simulink model "task4"  (R2018b)
settings: Solver=VariableStepAuto  StartTime=0.0  StopTime=5348  RelTol=1e-3
undefined symbols (not defined in the file): Ion, Lithium
libraries: powerlib x24, powerlib_meascontrol x6, electricdrivelib x4, pePwmGenerator x4, aerolibanimutils x1
settings Model: Creator=ibrahim yosry  LastModifiedBy=ibrahim yosry
settings SolverCC: ZeroCrossAlgorithm=Adaptive
settings DebuggingCC: IgnoredZcDiagnostic=none  LibraryContextMissingDiagnostic=none
settings SFSimCC: SimUseLocalCustomCode=off
settings RTWCC: RTWUseLocalCustomCode=off

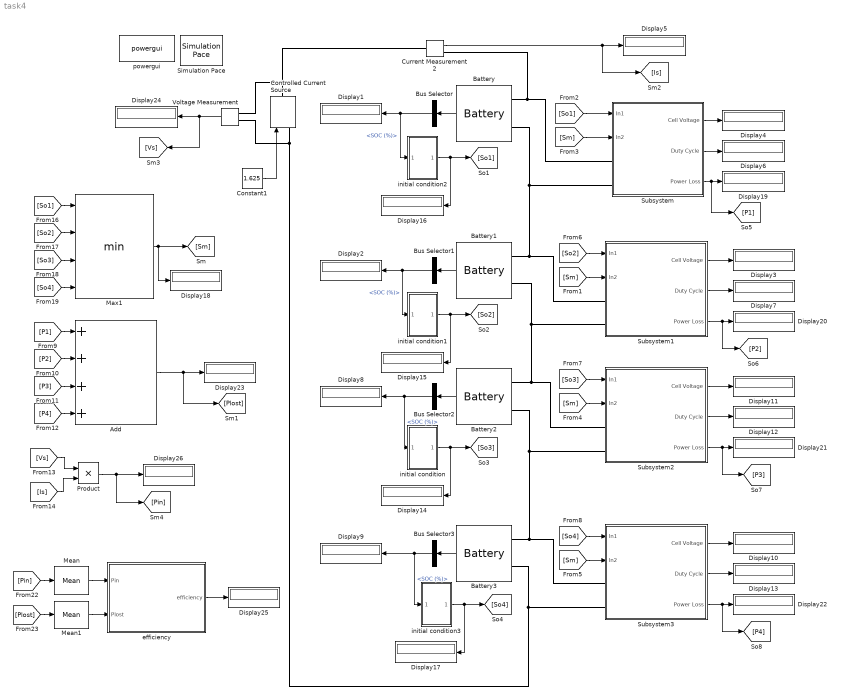
== system task4 ==
  Add : Sum  Inputs=++++
  Battery : electricdrivelib/Extra Sources/Battery  BatType=Lithium-Ion  ShowTempParam=off  ThermalPreset=no  ShowAgeParam=off  NomV=3.6  NomQ=3.4  SOC=14  Batt_Tr=30  PresetModel=on  MaxQ=3.4  MinV=2.7  FullV=4.1904  Dis_rate=1.4783  R=0.010588  Normal_OP=3.0748  expZone="[3.8894     0.16704]"  current=[6.5 13 32.5]  Units=Time  Tci=20  NomT=20  T2=-30  MaxQ2=4.8  FullV2=7.1  Normal_OP2=5.655  expZone2="[6.58           1]"  Rca=0.6  ti=2000  Dp=0  Neq0=0  Tsim=1e6  Ta1=25  Qeol=5.4*0.9  Reol=0.013333*1.2  Char_age=[2.3478, 3]  Dis_age=[2.3478, 10]  N1=1500  N2=10500  N3=1000  N4=1400  Ta2=45  N5=950
      settings: SourceProductName=Simscape Electrical
  Battery1 : electricdrivelib/Extra Sources/Battery  BatType=Lithium-Ion  ShowTempParam=off  ThermalPreset=no  ShowAgeParam=off  NomV=3.6  NomQ=3.4  SOC=24  Batt_Tr=30  PresetModel=on  MaxQ=3.4  MinV=2.7  FullV=4.1904  Dis_rate=1.4783  R=0.010588  Normal_OP=3.0748  expZone="[3.8894     0.16704]"  current=[6.5 13 32.5]  Units=Time  Tci=20  NomT=20  T2=-30  MaxQ2=4.8  FullV2=7.1  Normal_OP2=5.655  expZone2="[6.58           1]"  Rca=0.6  ti=2000  Dp=0  Neq0=0  Tsim=1e6  Ta1=25  Qeol=5.4*0.9  Reol=0.013333*1.2  Char_age=[2.3478, 3]  Dis_age=[2.3478, 10]  N1=1500  N2=10500  N3=1000  N4=1400  Ta2=45  N5=950
      settings: SourceProductName=Simscape Electrical
  Battery2 : electricdrivelib/Extra Sources/Battery  BatType=Lithium-Ion  ShowTempParam=off  ThermalPreset=no  ShowAgeParam=off  NomV=3.6  NomQ=3.4  SOC=30  Batt_Tr=30  PresetModel=on  MaxQ=3.4  MinV=2.7  FullV=4.1904  Dis_rate=1.4783  R=0.010588  Normal_OP=3.0748  expZone="[3.8894     0.16704]"  current=[6.5 13 32.5]  Units=Time  Tci=20  NomT=20  T2=-30  MaxQ2=4.8  FullV2=7.1  Normal_OP2=5.655  expZone2="[6.58           1]"  Rca=0.6  ti=2000  Dp=0  Neq0=0  Tsim=1e6  Ta1=25  Qeol=5.4*0.9  Reol=0.013333*1.2  Char_age=[2.3478, 3]  Dis_age=[2.3478, 10]  N1=1500  N2=10500  N3=1000  N4=1400  Ta2=45  N5=950
      settings: SourceProductName=Simscape Electrical
  Battery3 : electricdrivelib/Extra Sources/Battery  BatType=Lithium-Ion  ShowTempParam=off  ThermalPreset=no  ShowAgeParam=off  NomV=3.6  NomQ=3.4  SOC=45  Batt_Tr=30  PresetModel=on  MaxQ=3.4  MinV=2.7  FullV=4.1904  Dis_rate=1.4783  R=0.010588  Normal_OP=3.0748  expZone="[3.8894     0.16704]"  current=[6.5 13 32.5]  Units=Time  Tci=20  NomT=20  T2=-30  MaxQ2=4.8  FullV2=7.1  Normal_OP2=5.655  expZone2="[6.58           1]"  Rca=0.6  ti=2000  Dp=0  Neq0=0  Tsim=1e6  Ta1=25  Qeol=5.4*0.9  Reol=0.013333*1.2  Char_age=[2.3478, 3]  Dis_age=[2.3478, 10]  N1=1500  N2=10500  N3=1000  N4=1400  Ta2=45  N5=950
      settings: SourceProductName=Simscape Electrical
  Bus Selector{,1..3} (4 alike) : BusSelector  OutputSignals=SOC (%)
  Constant1 : Constant  Value=1.625
  Controlled Current Source : powerlib/Electrical Sources/Controlled Current Source  Initialize=on  Source_Type=DC  Amplitude=1.625  Phase=0  Frequency=0  Measurements=None
      settings: SourceProductName=Simscape Electrical
  Current Measurement2 : powerlib/Measurements/Current Measurement  PhasorSimulation=off  OutputType=Complex  PSBequivalent=0
      settings: SourceProductName=Simscape Electrical
  Display{1..26} (26 alike) : Display
  Max1 : MinMax  Inputs=4  ZeroCross=off
  Mean : powerlib_meascontrol/Measurements/Mean  Freq=1/1000  Vinit=0  Ts=0
  Mean1 : powerlib_meascontrol/Measurements/Mean  Freq=1/1000  Vinit=0  Ts=0
  Product : Product
  Simulation Pace : aerolibanimutils/Simulation Pace  SimulationPace=100  SleepMode=MATLAB Thread  OutputPaceError=off  SampleTime=1/30
  Subsystem : Subsystem
  Subsystem1 : Subsystem
  Subsystem2 : Subsystem
  Subsystem3 : Subsystem
  Voltage Measurement : powerlib/Measurements/Voltage Measurement  PhasorSimulation=off  OutputType=Complex  PSBequivalent=0
      settings: SourceProductName=Simscape Electrical
  efficiency : MATLAB Function  TreatAsAtomicUnit=on
  initial condition : Subsystem
      mask Display: image('F:\hima\zpEWIvRg.jpg');
  initial condition1 : Subsystem
      mask Display: image('F:\hima\zpEWIvRg.jpg');
  initial condition2 : Subsystem
      mask Display: image('F:\hima\zpEWIvRg.jpg');
  initial condition3 : Subsystem
      mask Display: image('F:\hima\zpEWIvRg.jpg');
  powergui : powerlib/powergui  Priority=1  SimulationMode=Continuous  SampleTime=50e-6  frequency=60  Iterations=50  frequencyindice=0  Pbase=100e6  ErrMax=1e-4  UnitsV=kV  UnitsW=MW  buscounter=0  FunctionMessages=off  echomessages=off  EnableUseOfTLC=off  CurrentSourceSwitches=off  DisableSnubberDevices=off  DisableRonSwitches=off  DisableVfSwitches=off  DisplayEquations=off  SolverType=Tustin/Backward Euler (TBE)  Interpol=off  ExternalGateDelay=off  methode=off  Ts=100  x0status=blocks  SPID=on  SwTol=0  HookPort=off  RestoreLinks=warning  ResistiveCurrentMeasurement=off  Frange=[0:2:500]  Ylog=off  Xlog=on  ShowGrid=off  save=off  variable=ZData  structure=0  ZoomFFT=off  StartTime=0.0  cycles=1  DisplayStyle=1  fundamental=60  FreqAxis=off  MaxFrequency=1000  frequencyindicesteady=1  RmsSteady=1  display=off
  wires:
  Bus Selector/1 -> initial condition2/1(<SOC (%)>), Display1/1  "<SOC (%)>"
  Constant1/1 -> Controlled Current Source/1
  Current Measurement2/1 -> [Is], Display5/1
  Battery/1 -> Bus Selector/1
  Subsystem/1(Cell Voltage) -> Display4/1
  Subsystem/2(Duty Cycle) -> Display6/1
  Subsystem1/1(Cell Voltage) -> Display3/1
  Subsystem1/2(Duty Cycle) -> Display7/1
  Battery1/1 -> Bus Selector1/1
  Bus Selector1/1 -> initial condition1/1(<SOC (%)>), Display2/1  "<SOC (%)>"
  Bus Selector3/1 -> initial condition3/1(<SOC (%)>), Display9/1  "<SOC (%)>"
  Subsystem2/2(Duty Cycle) -> Display12/1
  Subsystem3/1(Cell Voltage) -> Display10/1
  Battery3/1 -> Bus Selector3/1
  Subsystem2/1(Cell Voltage) -> Display11/1
  Subsystem3/2(Duty Cycle) -> Display13/1
  Battery2/1 -> Bus Selector2/1
  Bus Selector2/1 -> initial condition/1(<SOC (%)>), Display8/1  "<SOC (%)>"
  initial condition/1(Out1) -> [So3], Display14/1
  initial condition1/1(Out1) -> [So2], Display15/1
  initial condition2/1(Out1) -> [So1], Display16/1
  initial condition3/1(Out1) -> [So4], Display17/1
  [So2] -> Max1/2
  [So1] -> Max1/1
  Max1/1 -> [Sm], Display18/1
  [So3] -> Max1/3
  [So4] -> Max1/4
  [So1] -> Subsystem/1(In1)
  [Sm] -> Subsystem/2(In2)
  [Sm] -> Subsystem1/2(In2)
  [Sm] -> Subsystem2/2(In2)
  [Sm] -> Subsystem3/2(In2)
  [So2] -> Subsystem1/1(In1)
  [So3] -> Subsystem2/1(In1)
  [So4] -> Subsystem3/1(In1)
  Subsystem/3(Power Loss) -> Display19/1, [P1]
  Subsystem1/3(Power Loss) -> Display20/1, [P2]
  Subsystem2/3(Power Loss) -> Display21/1, [P3]
  Subsystem3/3(Power Loss) -> Display22/1, [P4]
  [P4] -> Add/4
  [P2] -> Add/2
  [P1] -> Add/1
  [P3] -> Add/3
  Voltage Measurement/1 -> Display24/1, [Vs]
  [Vs] -> Product/1
  [Is] -> Product/2
  efficiency/1(efficiency) -> Display25/1
  Product/1 -> Display26/1, [Pin]
  Add/1 -> Display23/1, [Plost]
  [Pin] -> Mean/1
  Mean/1 -> efficiency/1(Pin)
  Mean1/1 -> efficiency/2(Plost)
  [Plost] -> Mean1/1
  connections:
  Current Measurement2/LConn1 -- Controlled Current Source/RConn1 -- Voltage Measurement/LConn1
  Battery/LConn1 -- Current Measurement2/RConn1 -- Subsystem/LConn1
  Subsystem1/LConn1 -- Battery/LConn2 -- Subsystem/LConn2 -- Battery1/LConn1
  Subsystem2/LConn1 -- Battery1/LConn2 -- Subsystem1/LConn2 -- Battery2/LConn1
  Subsystem2/LConn2 -- Battery3/LConn1 -- Subsystem3/LConn1 -- Battery2/LConn2
  Subsystem3/LConn2 -- Controlled Current Source/LConn1 -- Voltage Measurement/LConn2 -- Battery3/LConn2

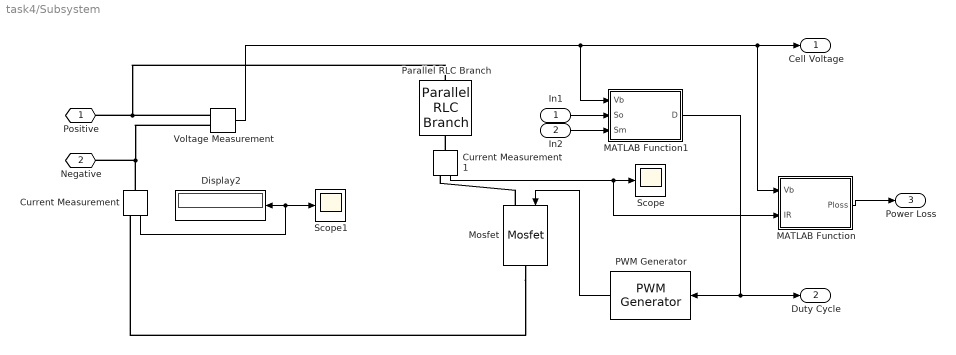
== system task4/Subsystem ==
  In1 : Inport
  In2 : Inport  Port=2
  Current Measurement : powerlib/Measurements/Current Measurement  PhasorSimulation=off  OutputType=Complex  PSBequivalent=0
      settings: SourceProductName=Simscape Electrical
  Current Measurement1 : powerlib/Measurements/Current Measurement  PhasorSimulation=off  OutputType=Complex  PSBequivalent=0
      settings: SourceProductName=Simscape Electrical
  Display2 : Display
  MATLAB Function : MATLAB Function  TreatAsAtomicUnit=on
  MATLAB Function1 : MATLAB Function  TreatAsAtomicUnit=on
  Mosfet : powerlib/Power Electronics/Mosfet  Ron=0.077  Lon=0  Rd=0.000000001  Vfd=0  IC=0  Rs=1e5  Cs=inf  Measurements=off
      settings: SourceProductName=Simscape Electrical
  PWM Generator : pePwmGenerator/PWM Generator  CarrCount=Up  Tper=1  Ts=0
  Parallel RLC Branch : powerlib/Elements/Parallel RLC Branch  LConnTagsString=a  RConnTagsString=__new0  BranchType=R  Resistance=2.7  Inductance=0  SetiL0=off  InitialCurrent=0  Capacitance=0  Setx0=off  InitialVoltage=0  Measurements=None
      settings: SourceProductName=Simscape Electrical
  Scope : Scope
  Scope1 : Scope
  Voltage Measurement : powerlib/Measurements/Voltage Measurement  PhasorSimulation=off  OutputType=Complex  PSBequivalent=0
      settings: SourceProductName=Simscape Electrical
  Positive : PMIOPort  Side=Left
  Negative : PMIOPort  Port=2  Side=Left
  Cell Voltage : Outport
  Duty Cycle : Outport  Port=2
  Power Loss : Outport  Port=3
  wires:
  MATLAB Function1/1(D) -> PWM Generator/1, Duty Cycle/1
  Current Measurement/1 -> Scope1/1, Display2/1
  Voltage Measurement/1 -> MATLAB Function/1(Vb), Cell Voltage/1, MATLAB Function1/1(Vb)
  PWM Generator/1 -> Mosfet/1
  Current Measurement1/1 -> MATLAB Function/2(IR), Scope/1
  In1/1 -> MATLAB Function1/2(So)
  In2/1 -> MATLAB Function1/3(Sm)
  MATLAB Function/1(Ploss) -> Power Loss/1
  connections:
  Current Measurement/LConn1 -- Voltage Measurement/LConn2 -- Negative/RConn1
  Mosfet/RConn1 -- Current Measurement/RConn1
  Current Measurement1/LConn1 -- Parallel RLC Branch/RConn1
  Mosfet/LConn1 -- Current Measurement1/RConn1
  Voltage Measurement/LConn1 -- Parallel RLC Branch/LConn1 -- Positive/RConn1

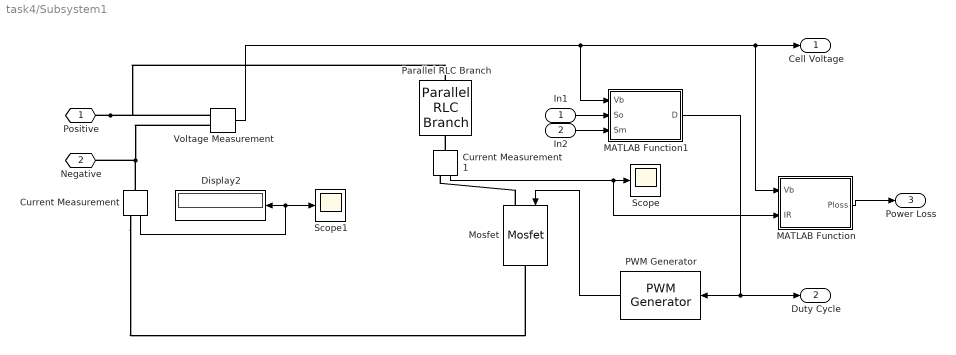
== system task4/Subsystem1 ==
  In1 : Inport
  In2 : Inport  Port=2
  Current Measurement : powerlib/Measurements/Current Measurement  PhasorSimulation=off  OutputType=Complex  PSBequivalent=0
      settings: SourceProductName=Simscape Electrical
  Current Measurement1 : powerlib/Measurements/Current Measurement  PhasorSimulation=off  OutputType=Complex  PSBequivalent=0
      settings: SourceProductName=Simscape Electrical
  Display2 : Display
  MATLAB Function : MATLAB Function  TreatAsAtomicUnit=on
  MATLAB Function1 : MATLAB Function  TreatAsAtomicUnit=on
  Mosfet : powerlib/Power Electronics/Mosfet  Ron=0.077  Lon=0  Rd=0.000000001  Vfd=0  IC=0  Rs=1e5  Cs=inf  Measurements=off
      settings: SourceProductName=Simscape Electrical
  PWM Generator : pePwmGenerator/PWM Generator  CarrCount=Up  Tper=1  Ts=0
  Parallel RLC Branch : powerlib/Elements/Parallel RLC Branch  LConnTagsString=a  RConnTagsString=__new0  BranchType=R  Resistance=2.7  Inductance=0  SetiL0=off  InitialCurrent=0  Capacitance=0  Setx0=off  InitialVoltage=0  Measurements=None
      settings: SourceProductName=Simscape Electrical
  Scope : Scope
  Scope1 : Scope
  Voltage Measurement : powerlib/Measurements/Voltage Measurement  PhasorSimulation=off  OutputType=Complex  PSBequivalent=0
      settings: SourceProductName=Simscape Electrical
  Positive : PMIOPort  Side=Left
  Negative : PMIOPort  Port=2  Side=Left
  Cell Voltage : Outport
  Duty Cycle : Outport  Port=2
  Power Loss : Outport  Port=3
  wires:
  MATLAB Function1/1(D) -> PWM Generator/1, Duty Cycle/1
  Current Measurement/1 -> Scope1/1, Display2/1
  Voltage Measurement/1 -> MATLAB Function/1(Vb), Cell Voltage/1, MATLAB Function1/1(Vb)
  PWM Generator/1 -> Mosfet/1
  Current Measurement1/1 -> MATLAB Function/2(IR), Scope/1
  In2/1 -> MATLAB Function1/3(Sm)
  In1/1 -> MATLAB Function1/2(So)
  MATLAB Function/1(Ploss) -> Power Loss/1
  connections:
  Voltage Measurement/LConn2 -- Current Measurement/LConn1 -- Negative/RConn1
  Current Measurement/RConn1 -- Mosfet/RConn1
  Current Measurement1/LConn1 -- Parallel RLC Branch/RConn1
  Mosfet/LConn1 -- Current Measurement1/RConn1
  Positive/RConn1 -- Voltage Measurement/LConn1 -- Parallel RLC Branch/LConn1

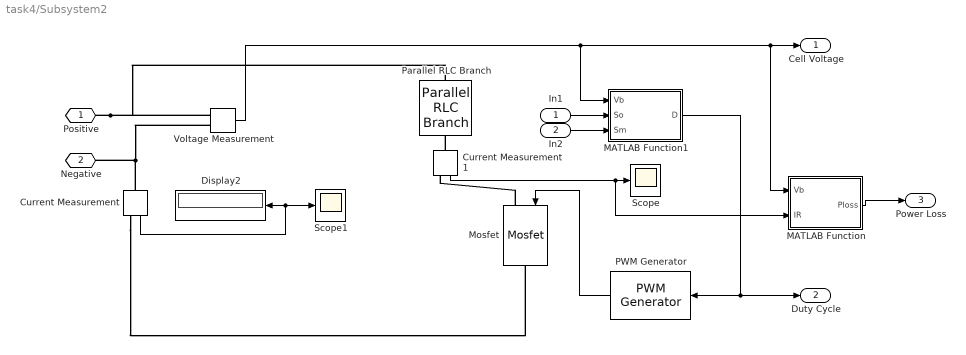
== system task4/Subsystem2 ==
  In1 : Inport
  In2 : Inport  Port=2
  Current Measurement : powerlib/Measurements/Current Measurement  PhasorSimulation=off  OutputType=Complex  PSBequivalent=0
      settings: SourceProductName=Simscape Electrical
  Current Measurement1 : powerlib/Measurements/Current Measurement  PhasorSimulation=off  OutputType=Complex  PSBequivalent=0
      settings: SourceProductName=Simscape Electrical
  Display2 : Display
  MATLAB Function : MATLAB Function  TreatAsAtomicUnit=on
  MATLAB Function1 : MATLAB Function  TreatAsAtomicUnit=on
  Mosfet : powerlib/Power Electronics/Mosfet  Ron=0.077  Lon=0  Rd=0.000000001  Vfd=0  IC=0  Rs=1e5  Cs=inf  Measurements=off
      settings: SourceProductName=Simscape Electrical
  PWM Generator : pePwmGenerator/PWM Generator  CarrCount=Up  Tper=1  Ts=0
  Parallel RLC Branch : powerlib/Elements/Parallel RLC Branch  LConnTagsString=a  RConnTagsString=__new0  BranchType=R  Resistance=2.7  Inductance=0  SetiL0=off  InitialCurrent=0  Capacitance=0  Setx0=off  InitialVoltage=0  Measurements=None
      settings: SourceProductName=Simscape Electrical
  Scope : Scope
  Scope1 : Scope
  Voltage Measurement : powerlib/Measurements/Voltage Measurement  PhasorSimulation=off  OutputType=Complex  PSBequivalent=0
      settings: SourceProductName=Simscape Electrical
  Positive : PMIOPort  Side=Left
  Negative : PMIOPort  Port=2  Side=Left
  Cell Voltage : Outport
  Duty Cycle : Outport  Port=2
  Power Loss : Outport  Port=3
  wires:
  MATLAB Function1/1(D) -> PWM Generator/1, Duty Cycle/1
  Current Measurement/1 -> Scope1/1, Display2/1
  Voltage Measurement/1 -> MATLAB Function/1(Vb), Cell Voltage/1, MATLAB Function1/1(Vb)
  PWM Generator/1 -> Mosfet/1
  Current Measurement1/1 -> MATLAB Function/2(IR), Scope/1
  In2/1 -> MATLAB Function1/3(Sm)
  In1/1 -> MATLAB Function1/2(So)
  MATLAB Function/1(Ploss) -> Power Loss/1
  connections:
  Voltage Measurement/LConn2 -- Current Measurement/LConn1 -- Negative/RConn1
  Current Measurement/RConn1 -- Mosfet/RConn1
  Current Measurement1/LConn1 -- Parallel RLC Branch/RConn1
  Mosfet/LConn1 -- Current Measurement1/RConn1
  Positive/RConn1 -- Voltage Measurement/LConn1 -- Parallel RLC Branch/LConn1

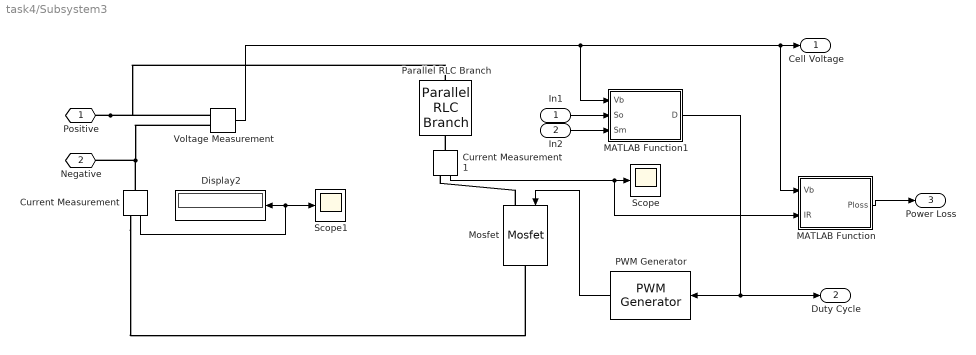
== system task4/Subsystem3 ==
  In1 : Inport
  In2 : Inport  Port=2
  Current Measurement : powerlib/Measurements/Current Measurement  PhasorSimulation=off  OutputType=Complex  PSBequivalent=0
      settings: SourceProductName=Simscape Electrical
  Current Measurement1 : powerlib/Measurements/Current Measurement  PhasorSimulation=off  OutputType=Complex  PSBequivalent=0
      settings: SourceProductName=Simscape Electrical
  Display2 : Display
  MATLAB Function : MATLAB Function  TreatAsAtomicUnit=on
  MATLAB Function1 : MATLAB Function  TreatAsAtomicUnit=on
  Mosfet : powerlib/Power Electronics/Mosfet  Ron=0.077  Lon=0  Rd=0.000000001  Vfd=0  IC=0  Rs=1e5  Cs=inf  Measurements=off
      settings: SourceProductName=Simscape Electrical
  PWM Generator : pePwmGenerator/PWM Generator  CarrCount=Up  Tper=1  Ts=0
  Parallel RLC Branch : powerlib/Elements/Parallel RLC Branch  LConnTagsString=a  RConnTagsString=__new0  BranchType=R  Resistance=2.7  Inductance=0  SetiL0=off  InitialCurrent=0  Capacitance=0  Setx0=off  InitialVoltage=0  Measurements=None
      settings: SourceProductName=Simscape Electrical
  Scope : Scope
  Scope1 : Scope
  Voltage Measurement : powerlib/Measurements/Voltage Measurement  PhasorSimulation=off  OutputType=Complex  PSBequivalent=0
      settings: SourceProductName=Simscape Electrical
  Positive : PMIOPort  Side=Left
  Negative : PMIOPort  Port=2  Side=Left
  Cell Voltage : Outport
  Duty Cycle : Outport  Port=2
  Power Loss : Outport  Port=3
  wires:
  MATLAB Function1/1(D) -> PWM Generator/1, Duty Cycle/1
  Current Measurement/1 -> Scope1/1, Display2/1
  Voltage Measurement/1 -> MATLAB Function/1(Vb), Cell Voltage/1, MATLAB Function1/1(Vb)
  PWM Generator/1 -> Mosfet/1
  Current Measurement1/1 -> MATLAB Function/2(IR), Scope/1
  In2/1 -> MATLAB Function1/3(Sm)
  In1/1 -> MATLAB Function1/2(So)
  MATLAB Function/1(Ploss) -> Power Loss/1
  connections:
  Voltage Measurement/LConn2 -- Current Measurement/LConn1 -- Negative/RConn1
  Current Measurement/RConn1 -- Mosfet/RConn1
  Current Measurement1/LConn1 -- Parallel RLC Branch/RConn1
  Mosfet/LConn1 -- Current Measurement1/RConn1
  Positive/RConn1 -- Voltage Measurement/LConn1 -- Parallel RLC Branch/LConn1

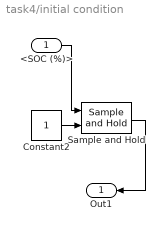
== system task4/initial condition ==
  <SOC (%)> : Inport
  Constant2 : Constant
  Sample and Hold : powerlib_meascontrol/Additional Components/Sample and Hold  ic=0  Ts=6000000
      settings: SourceProductName=Simscape Power Systems  SourceProductBaseCode=PS
  Out1 : Outport
  wires:
  Constant2/1 -> Sample and Hold/2
  <SOC (%)>/1 -> Sample and Hold/1
  Sample and Hold/1 -> Out1/1

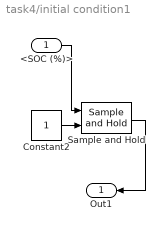
== system task4/initial condition1 ==
  <SOC (%)> : Inport
  Constant2 : Constant
  Sample and Hold : powerlib_meascontrol/Additional Components/Sample and Hold  ic=0  Ts=6000000
      settings: SourceProductName=Simscape Power Systems  SourceProductBaseCode=PS
  Out1 : Outport
  wires:
  Constant2/1 -> Sample and Hold/2
  <SOC (%)>/1 -> Sample and Hold/1
  Sample and Hold/1 -> Out1/1

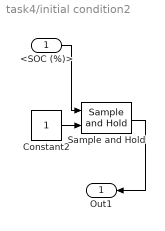
== system task4/initial condition2 ==
  <SOC (%)> : Inport
  Constant2 : Constant
  Sample and Hold : powerlib_meascontrol/Additional Components/Sample and Hold  ic=0  Ts=6000000
      settings: SourceProductName=Simscape Power Systems  SourceProductBaseCode=PS
  Out1 : Outport
  wires:
  Constant2/1 -> Sample and Hold/2
  <SOC (%)>/1 -> Sample and Hold/1
  Sample and Hold/1 -> Out1/1

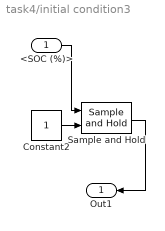
== system task4/initial condition3 ==
  <SOC (%)> : Inport
  Constant2 : Constant
  Sample and Hold : powerlib_meascontrol/Additional Components/Sample and Hold  ic=0  Ts=6000000
      settings: SourceProductName=Simscape Power Systems  SourceProductBaseCode=PS
  Out1 : Outport
  wires:
  Constant2/1 -> Sample and Hold/2
  <SOC (%)>/1 -> Sample and Hold/1
  Sample and Hold/1 -> Out1/1

== matlab function task4/Subsystem/MATLAB Function1 ==
  data: Vb input; D output; So input; Sm input
function D = fcn(Vb,So,Sm)
Sf=85;
It=1.625;
R=2.777;
D = (It*R/Vb)*(So/100-Sm/100)/(Sf/100-Sm/100);

== matlab function task4/Subsystem/MATLAB Function ==
  data: Vb input; Ploss output; IR input
function Ploss = fcn(Vb,IR)
R=2.777;
f=1;
Ploss =((IR^2)*R)+((75.5e-9)*f*(Vb^2)/R);

== matlab function task4/Subsystem1/MATLAB Function ==
  data: Vb input; Ploss output; IR input
function Ploss = fcn(Vb,IR)
R=2.777;
f=1;
Ploss =((IR^2)*R)+((75.5e-9)*f*(Vb^2)/R);

== matlab function task4/Subsystem1/MATLAB Function1 ==
  data: Vb input; D output; So input; Sm input
function D = fcn(Vb,So,Sm)
Sf=85;
It=1.625;
R=2.777;
D = (It*R/Vb)*(So/100-Sm/100)/(Sf/100-Sm/100);

== matlab function task4/Subsystem2/MATLAB Function ==
  data: Vb input; Ploss output; IR input
function Ploss = fcn(Vb,IR)
R=2.777;
f=1;
Ploss =((IR^2)*R)+((75.5e-9)*f*(Vb^2)/R);

== matlab function task4/Subsystem2/MATLAB Function1 ==
  data: Vb input; D output; So input; Sm input
function D = fcn(Vb,So,Sm)
Sf=85;
It=1.625;
R=2.777;
D = (It*R/Vb)*(So/100-Sm/100)/(Sf/100-Sm/100);

== matlab function task4/Subsystem3/MATLAB Function ==
  data: Vb input; Ploss output; IR input
function Ploss = fcn(Vb,IR)
R=2.777;
f=1;
Ploss =((IR^2)*R)+((75.5e-9)*f*(Vb^2)/R);

== matlab function task4/Subsystem3/MATLAB Function1 ==
  data: Vb input; D output; So input; Sm input
function D = fcn(Vb,So,Sm)
Sf=85;
It=1.625;
R=2.777;
D = (It*R/Vb)*(So/100-Sm/100)/(Sf/100-Sm/100);

== matlab function task4/efficiency ==
  data: Pin input; efficiency output; Plost input
function efficiency = fcn(Pin,Plost)

efficiency = ((Pin-Plost)/Pin)*100;
